simulink model "dynamic_eular"  (R2025a)
settings: Solver=VariableStepAuto  StartTime=0.0  StopTime=10.0  RelTol=1e-3
settings Model: Creator=rlwan  LastModifiedBy=rlwan

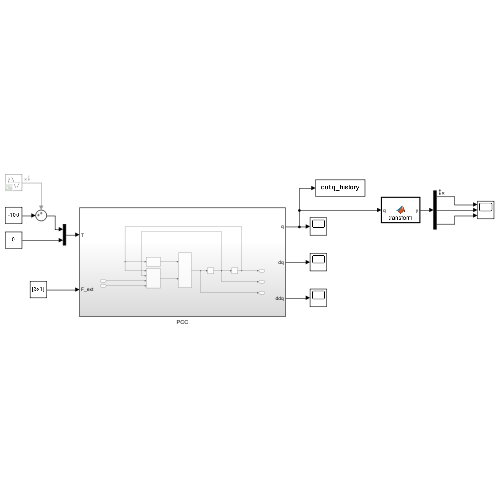
[thumbnail: Simulink's stored preview of the top-level diagram]
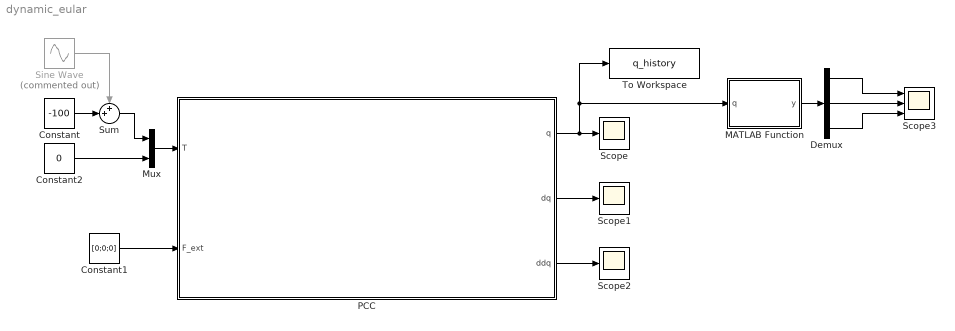
== system dynamic_eular ==
  Constant : Constant  Value=-100
  Constant1 : Constant  Value=[0;0;0]
  Constant2 : Constant  Value=0
  Demux : Demux  Outputs=3
  MATLAB Function : MATLAB Function  TreatAsAtomicUnit=on
  Mux : Mux  Inputs=2
  PCC : Subsystem
  Scope : Scope
      settings: ActiveDisplayYMinimum=-0.073811965831007964  ActiveDisplayYMaximum=0.59923738312001884
  Scope1 : Scope
      settings: ActiveDisplayYMinimum=-1.2562951553581858  ActiveDisplayYMaximum=1.3493657939233712
  Scope2 : Scope
      settings: ActiveDisplayYMinimum=-3.5396008111253705  ActiveDisplayYMaximum=2.911379815977388  DataLoggingVariableName=ScopeData2
  Scope3 : Scope  NumInputPorts=3
      settings: ActiveDisplayYMinimum=-0.31972307217971685  ActiveDisplayYMaximum=1.2379856473633313  DataLoggingVariableName=ScopeData3
  Sine Wave : Sin  Commented=on  SampleTime=0
  Sum : Sum  Inputs=++|
  To Workspace : ToWorkspace  VariableName=q_history  SampleTime=-1
  wires:
  Constant1/1 -> PCC/2(F_ext)
  PCC/3(ddq) -> Scope2/1
  Mux/1 -> PCC/1(T)
  Sine Wave/1 -> Sum/1
  MATLAB Function/1(y) -> Demux/1
  PCC/2(dq) -> Scope1/1
  Demux/2 -> Scope3/2
  PCC/1(q) -> To Workspace/1, MATLAB Function/1(q), Scope/1
  Constant2/1 -> Mux/2
  Demux/1 -> Scope3/1
  Demux/3 -> Scope3/3
  Constant/1 -> Sum/2
  Sum/1 -> Mux/1

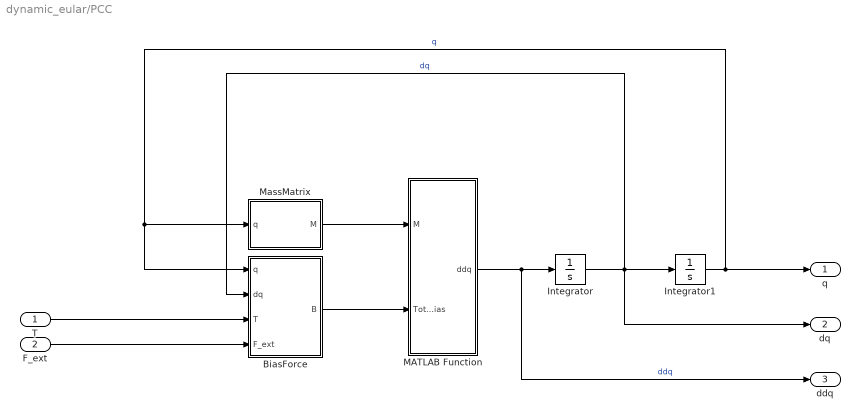
== system dynamic_eular/PCC ==
  T : Inport
  F_ext : Inport  Port=2
  BiasForce : MATLAB Function  TreatAsAtomicUnit=on
  Integrator : Integrator  InitialCondition=zeros(4,1)
  Integrator1 : Integrator  InitialCondition=zeros(4,1)
  MATLAB Function : MATLAB Function  TreatAsAtomicUnit=on
  MassMatrix : MATLAB Function  TreatAsAtomicUnit=on
  q : Outport
  dq : Outport  Port=2
  ddq : Outport  Port=3
  wires:
  T/1 -> BiasForce/3(T)
  BiasForce/1(B) -> MATLAB Function/2(TotalBias)
  MassMatrix/1(M) -> MATLAB Function/1(M)
  MATLAB Function/1(ddq) -> ddq/1, Integrator/1  "ddq"
  Integrator1/1 -> q/1, BiasForce/1(q), MassMatrix/1(q)  "q"
  F_ext/1 -> BiasForce/4(F_ext)
  Integrator/1 -> dq/1, BiasForce/2(dq), Integrator1/1  "dq"

== matlab function dynamic_eular/PCC/BiasForce ==
  data: q input; B output; dq input; T input; F_ext input
function B = fcn(q, dq, T, F_ext)

Tx = T(1); Ty = T(2);
fx = F_ext(1); fy = F_ext(2); fz = F_ext(3);

GKForce = get_GKForce_Euler(q);
DampForce = get_DampForce_Euler(dq);
ExtForce = get_ExtForce_Euler(q, dq, Tx, Ty, fx, fy, fz);
B = GKForce+DampForce+ExtForce;

% EPSILON_THETA = 1e-3;
% 
% if q(1) < EPSILON_THETA
%     q(1) = EPSILON_THETA;
% end
% if q(4) < EPSILON_THETA
%     q(4) = EPSILON_THETA;
% end
% 
% CoriolisForce = get_Coriolis(q, dq);
% 
% B = B + CoriolisForce;

== matlab function dynamic_eular/PCC/MassMatrix ==
  data: q input; M output
function M = fcn(q)

M = get_MassMatrix_Euler(q);

== matlab function dynamic_eular/PCC/MATLAB Function ==
  data: M input; ddq output; TotalBias input
function ddq = Solver(M, TotalBias)

    M_stable = M + eye(size(M)) * 1e-5;

    ddq = M_stable \ (-TotalBias);
    
    limit = 1e3;
    ddq = max(min(ddq, limit), -limit);
end

== matlab function dynamic_eular/MATLAB Function ==
  data: q input; y output
function y = transform(q)

N = 2; % PCC段数

H_0 = get_homogeneous_Euler(q);
y = H_0(1:3,4,N);
